simulink model "DTMF_DSK6713"  (Simulink 6.5)
settings: Solver=FixedStepDiscrete  StartTime=0  StopTime=20  RelTol=1e-3
PreLoadFcn:
  | Framesize=256,Fs=8192
values from neighbouring files (symbols this model uses):
  x = single(get(hObject,'Value'))    [AM.m]
undefined symbols (not defined in the file or in its folder): bit, dfilt, Fs
libraries: dspddes3 x14, dspobslib x3, commutil2 x2, c6713dsklib x1, c6000tgtpreflib x1, dsparch3 x1, dspswit3 x1, dspbuff3 x1, dsparch4 x1, rtdxBlocks x1
settings Model: Creator=stuartm  LastModifiedBy=dsp  ExtModeTrigMode=oneshot  ExtModeArmWhenConnect=off  BufferReuse=off  ProdHWDeviceType=TI C6000
settings SolverCC: PositivePriorityOrder=on
settings DataIOCC: LimitDataPoints=off  SaveOutput=off  SaveTime=off  SignalLoggingName=sigsOut
settings OptimizationCC: BlockReduction=off  BooleanDataType=off  OptimizeBlockIOStorage=off  BufferReuse=off  EnforceIntegerDowncast=off  ExpressionFolding=off  FoldNonRolledExpr=off  LocalBlockOutputs=off  OptimizeModelRefInitCode=on
settings DebuggingCC: SolverPrmCheckMsg=none  MultiTaskDSMMsg=warning  MultiTaskCondExecSysMsg=none  StrictBusMsg=None
settings HardwareCC: ProdBitPerLong=40  ProdIntDivRoundTo=Zero  ProdEndianess=LittleEndian  ProdHWDeviceType=TI C6000
settings RTWCC: SystemTargetFile=ti_c6000_ert.tlc  GenCodeOnly=on  TemplateMakefile=ti_c6000_ert.tmf  Description=Embedded Target for TI C6000 DSP (ERT)  ProcessScript=ti_c6000_ert_make_rtw_hook  IncludeERTFirstTime=on
settings CodeAppCC: IgnoreCustomStorageClasses=off
settings C6000ERTTargetCC: TargetFcnLib=ansi_tfl_tmw.mat  GenFloatMathFcnCalls=ANSI_C  UtilityFuncGeneration=Auto  GenerateFullHeader=on  GenerateSampleERTMain=off  GenerateTestInterfaces=off  IsPILTarget=off  ModelReferenceCompliant=on  IncludeMdlTerminateFcn=on  CombineOutputUpdateFcns=on  SuppressErrorStatus=off  IncludeFileDelimiter=Auto  ERTCustomFileBanners=on  SupportAbsoluteTime=on  LogVarNameModifier=rt_  MatFileLogging=off  MultiInstanceERTCode=off  SupportNonFinite=on  SupportComplex=on  PurelyIntegerCode=off  SupportContinuousTime=off  SupportNonInlinedSFcns=off  EnableShiftOperators=on  ParenthesesLevel=Nominal  GenerateErtSFunction=off  GenerateASAP2=off  ExtMode=off  ExtModeTransport=0  ExtModeStaticAlloc=off  ExtModeStaticAllocSize=1000000  ExtModeTesting=off  ExtModeMexFile=ext_comm  InlinedParameterPlacement=NonHierarchical  TargetOS=BareBoardExample  MultiInstanceErrorCode=Error  RateGroupingCode=on  RootIOFormat=Individual arguments  RTWCAPISignals=off  RTWCAPIParams=off  RTWCAPIStates=off  ERTSrcFileBannerTemplate=ert_code_template.cgt  ERTHdrFileBannerTemplate=ert_code_template.cgt  ERTDataSrcFileTemplate=ert_code_template.cgt  ERTDataHdrFileTemplate=ert_code_template.cgt  ERTCustomFileTemplate=example_file_process.tlc  ModuleNamingRule=Unspecified  SignalDisplayLevel=10  ParamTuneLevel=10  GlobalDataDefinition=Auto  DataDefinitionFile=global.c  GlobalDataReference=Auto  DataReferenceFile=global.h  GRTInterface=off  EnableUserReplacementTypes=off  MemSecPackage=--- None ---  MemSecDataConstants=Default  MemSecDataIO=Default  MemSecDataInternal=Default  MemSecDataParameters=Default  MemSecFuncInitTerm=Default  MemSecFuncExecute=Default  exportCCSObj=on  ccsObjName=CCS_Obj  useDSPBIOS=on  ProfileGenCode=on  InlineDSPBlks=on  FPopt=off  memModel=Far_Aggregate  optLevel=Function(-o2)  CompilerVerbosity=Quiet  InterruptThreshOnC6x=off  SymbolicDebugOnC6x=off  RetainAsmFiles=off  RetainObjFiles=on  CreateMapFile=on  UserStackSize=8192  c6000BuildAction=Build  OverrunAction=Notify_and_continue  OverrunNotificationMethod=Turn_on_LEDs

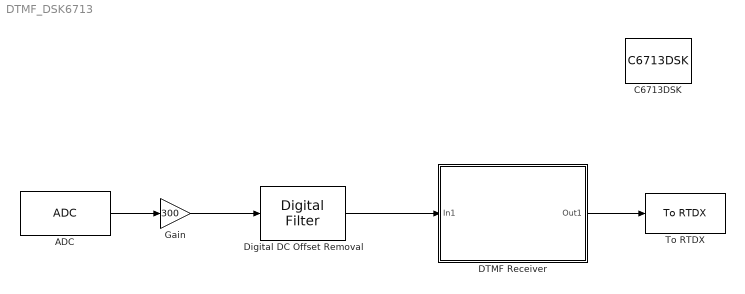
== system DTMF_DSK6713 ==
  ADC : c6713dsklib/ADC  ADCsource=Line In  MicGain=off  Stereo=off  SampleRate=8 kHz  CodecDataFormat=16-bit  OutputDataType=Double  Scaling=Normalize  SourceGain=0.0  FrameSize=256  inheritSampleTime=off
  C6713DSK : c6000tgtpreflib/C6713DSK  Tag=C6000 TARGET PREFERENCES BLOCK  SystemSampleTime=-1
  DTMF Receiver : Subsystem
  Digital DC Offset Removal : dsparch4/Digital Filter  DialogController=dspdialog.DigitalFilter  DialogControllerArgs=DataTag1  TypePopup=FIR (all zeros)  IIRFiltStruct=Direct form II transposed  AllPoleFiltStruct=Direct form  FIRFiltStruct=Direct form  CoeffSource=Specify via dialog  NumCoeffs=[0.5 -0.5]  DenCoeffs=[1 0.1]  BiQuadCoeffs=[1 0.3 0.4 1 0.1 0.2]  LatticeCoeffs=[0.2 0.4]  denIgnore=on  FiltPerSampPopup=One filter per frame  IC=0  ICnum=0  ICden=0  roundingMode=Floor  overflowMode=off  ScaleValues=1  scaleValueFracLength=14  stageInFracLength=15  stageOutFracLength=15  FilterSource=Specify via dialog  dfiltObjectName=dfilt.dffir([1 2 1])
  Gain : Gain  Gain=300
  To RTDX : rtdxBlocks/To RTDX  channelNameStr=OutputDigit  isBlocking=on  isChannelEnabled=on
  wires:
  Digital DC Offset Removal/1 -> DTMF Receiver/1(In1)
  DTMF Receiver/1(Out1) -> To RTDX/1
  Gain/1 -> Digital DC Offset Removal/1
  ADC/1 -> Gain/1

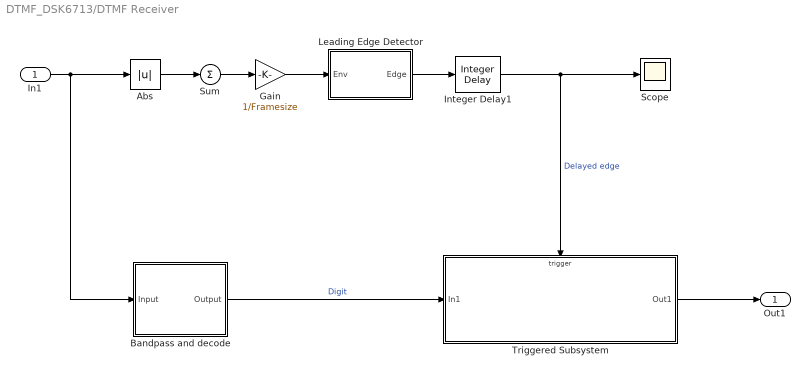
== system DTMF_DSK6713/DTMF Receiver ==
  In1 : Inport
  Abs : Abs  SaturateOnIntegerOverflow=on  SampleTime=-1
  Bandpass and decode : Subsystem
  Gain : Gain  Gain=1/Framesize  SaturateOnIntegerOverflow=on
  Integer Delay1 : dspobslib/Integer Delay  delay=1  ic=0  reset_popup=None
  Leading Edge Detector : Subsystem
  Scope : Scope
  Sum : Sum  Inputs=1  SaturateOnIntegerOverflow=on  InputSameDT=on
  Triggered Subsystem : Subsystem  TreatAsAtomicUnit=on
  Out1 : Outport
  wires:
  In1/1 -> Abs/1, Bandpass and decode/1(Input)
  Abs/1 -> Sum/1
  Sum/1 -> Gain/1
  Gain/1 -> Leading Edge Detector/1(Env)
  Triggered Subsystem/1(Out1) -> Out1/1
  Integer Delay1/1 -> Scope/1, Triggered Subsystem/Trigger  "Delayed edge"
  Bandpass and decode/1(Output) -> Triggered Subsystem/1(In1)  "Digit"
  Leading Edge Detector/1(Edge) -> Integer Delay1/1

== system DTMF_DSK6713/DTMF Receiver/Bandpass and decode ==
  Input : Inport
  Calculate Digit : Lookup2D  RowIndex=[1:4]  ColumnIndex=[1:3]  OutputValues=[1 2 3;4 5 6;7 8 9;10 0 11]  LookUpMeth=Use Input Nearest  OutDataTypeMode=double  SaturateOnIntegerOverflow=on  InputSameDT=on
  Calculate Column : Subsystem
  Calculate Row : Subsystem
  Output : Outport
  wires:
  Input/1 -> Calculate Column/1(In1), Calculate Row/1(In1)  "Input Tones"
  Calculate Digit/1 -> Output/1
  Calculate Row/1(Out1) -> Calculate Digit/1
  Calculate Column/1(Out1) -> Calculate Digit/2

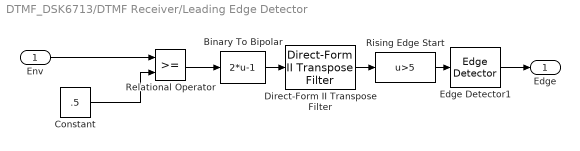
== system DTMF_DSK6713/DTMF Receiver/Leading Edge Detector ==
  Env : Inport
  Binary To Bipolar : Fcn  Expr=2*u-1
  Constant : Constant  Value=.5  OutDataType=sfix(16)  ConRadixGroup=Use specified scaling  OutScaling=2^0  SampleTime=inf  FramePeriod=inf
  Direct-Form II Transpose Filter : dsparch3/Direct-Form II Transpose Filter  num=[ones(1,4) -ones(1,4)]  den=1  ic=0
  Edge Detector1 : dspswit3/Edge Detector  SystemSampleTime=-1
  Relational Operator : RelationalOperator  InputSameDT=on
  Rising Edge Start : Fcn  Expr=u>5
  Edge : Outport  InitialOutput=0
  wires:
  Edge Detector1/1 -> Edge/1
  Direct-Form II Transpose Filter/1 -> Rising Edge Start/1
  Binary To Bipolar/1 -> Direct-Form II Transpose Filter/1
  Rising Edge Start/1 -> Edge Detector1/1
  Env/1 -> Relational Operator/1
  Constant/1 -> Relational Operator/2
  Relational Operator/1 -> Binary To Bipolar/1

== system DTMF_DSK6713/DTMF Receiver/Triggered Subsystem ==
  In1 : Inport
  Trigger : TriggerPort
  Buffer : dspbuff3/Buffer  N=11  V=10  ic=0
  Out1 : Outport
  wires:
  In1/1 -> Buffer/1
  Buffer/1 -> Out1/1

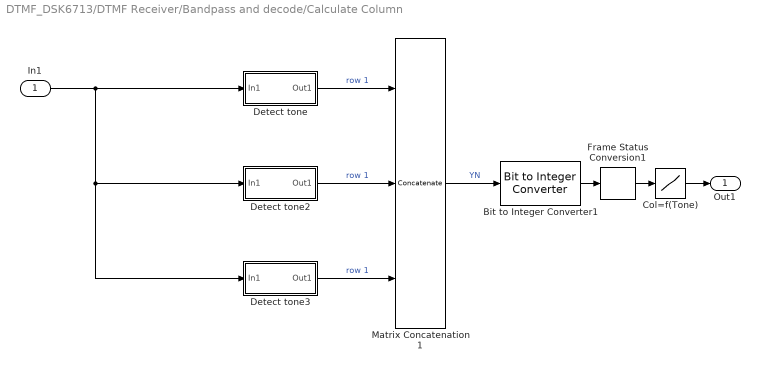
== system DTMF_DSK6713/DTMF Receiver/Bandpass and decode/Calculate Column ==
  In1 : Inport
  Bit to Integer Converter1 : commutil2/Bit to Integer Converter  nbits=3  outDtype=Same as input
  Col=f(Tone) : Lookup  InputValues=[0:7]  OutputValues=[0 1 2 0 3 0 0 0]  LookUpMeth=Use Input Nearest  OutDataType=sfix(16)  OutScaling=2^0  SaturateOnIntegerOverflow=on  SampleTime=-1  LUTDesignTableMode=Redesign Table  LUTDesignDataSource=Block Dialog  LUTDesignFunctionName=sqrt(x)  LUTDesignUseExistingBP=on  LUTDesignRelError=0.01  LUTDesignAbsError=1e-6  RndMeth=Floor
      settings: LockScale=off
  Detect tone : Subsystem  mask{Fs=Fs, F=1477}
      mask prompts: Fs "Sample Rate (Hz)"; F "Frequency"
      settings: AttributesFormatString=%<F> Hz
  Detect tone2 : Subsystem  mask{Fs=Fs, F=1336}
      mask prompts: Fs "Sample Rate (Hz)"; F "Frequency"
      settings: AttributesFormatString=%<F> Hz
  Detect tone3 : Subsystem  mask{Fs=Fs, F=1209}
      mask prompts: Fs "Sample Rate (Hz)"; F "Frequency"
      settings: AttributesFormatString=%<F> Hz
  Frame Status Conversion1 : dspobslib/Frame Status Conversion  SystemSampleTime=-1  growRefPort=off  outframe=Sample-based
  Matrix Concatenation1 : Concatenate  NumInputs=3  Mode=Vertical matrix concatenation
  Out1 : Outport
  wires:
  Matrix Concatenation1/1 -> Bit to Integer Converter1/1  "YN"
  Bit to Integer Converter1/1 -> Frame Status Conversion1/1
  Frame Status Conversion1/1 -> Col=f(Tone)/1
  Detect tone/1(Out1) -> Matrix Concatenation1/1  "row 1"
  Detect tone2/1(Out1) -> Matrix Concatenation1/2  "row 1"
  Detect tone3/1(Out1) -> Matrix Concatenation1/3  "row 1"
  In1/1 -> Detect tone2/1(In1), Detect tone3/1(In1), Detect tone/1(In1)
  Col=f(Tone)/1 -> Out1/1

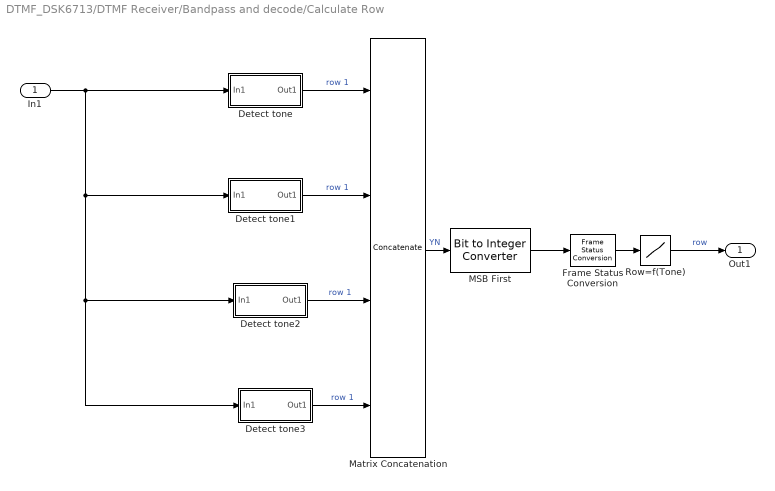
== system DTMF_DSK6713/DTMF Receiver/Bandpass and decode/Calculate Row ==
  In1 : Inport
  Detect tone : Subsystem  mask{Fs=Fs, F=941}
      mask prompts: Fs "Sample Rate (Hz)"; F "Frequency"
      settings: AttributesFormatString=%<F> Hz
  Detect tone1 : Subsystem  mask{Fs=Fs, F=852}
      mask prompts: Fs "Sample Rate (Hz)"; F "Frequency"
      settings: AttributesFormatString=%<F> Hz
  Detect tone2 : Subsystem  mask{Fs=Fs, F=770}
      mask prompts: Fs "Sample Rate (Hz)"; F "Frequency"
      settings: AttributesFormatString=%<F> Hz
  Detect tone3 : Subsystem  mask{Fs=Fs, F=697}
      mask prompts: Fs "Sample Rate (Hz)"; F "Frequency"
      settings: AttributesFormatString=%<F> Hz
  Frame Status Conversion : dspobslib/Frame Status Conversion  SystemSampleTime=-1  growRefPort=off  outframe=Sample-based
  MSB First : commutil2/Bit to Integer Converter  nbits=4  outDtype=Same as input
  Matrix Concatenation : Concatenate  NumInputs=4  Mode=Vertical matrix concatenation
  Row=f(Tone) : Lookup  InputValues=[0:15]  OutputValues=[0 1 2 0 3 0 0 0 4 0 0 0 0 0 0 0]  LookUpMeth=Use Input Nearest  OutDataType=sfix(16)  OutScaling=2^0  SaturateOnIntegerOverflow=on  SampleTime=-1  LUTDesignTableMode=Redesign Table  LUTDesignDataSource=Block Dialog  LUTDesignFunctionName=sqrt(x)  LUTDesignUseExistingBP=on  LUTDesignRelError=0.01  LUTDesignAbsError=1e-6  RndMeth=Floor
      settings: LockScale=off
  Out1 : Outport
  wires:
  Detect tone/1(Out1) -> Matrix Concatenation/1  "row 1"
  Matrix Concatenation/1 -> MSB First/1  "YN"
  MSB First/1 -> Frame Status Conversion/1
  Frame Status Conversion/1 -> Row=f(Tone)/1
  Detect tone1/1(Out1) -> Matrix Concatenation/2  "row 1"
  Detect tone2/1(Out1) -> Matrix Concatenation/3  "row 1"
  Detect tone3/1(Out1) -> Matrix Concatenation/4  "row 1"
  In1/1 -> Detect tone/1(In1), Detect tone1/1(In1), Detect tone2/1(In1), Detect tone3/1(In1)
  Row=f(Tone)/1 -> Out1/1  "row"

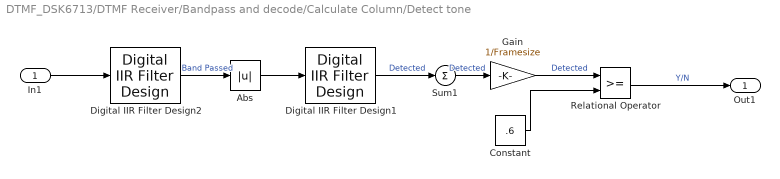
== system DTMF_DSK6713/DTMF Receiver/Bandpass and decode/Calculate Column/Detect tone ==
  In1 : Inport
  Abs : Abs  SaturateOnIntegerOverflow=on  SampleTime=-1
  Constant : Constant  Value=.6  OutDataType=sfix(16)  ConRadixGroup=Use specified scaling  OutScaling=2^0  SampleTime=inf  FramePeriod=inf
  Digital IIR Filter Design1 : dspddes3/Digital IIR Filter Design  SystemSampleTime=-1  method=Butterworth  filttype=Lowpass  N=4  Wlo=100/(Fs/2)  Whi=(F+10)/(Fs/2)  Rp=1  Rs=20
  Digital IIR Filter Design2 : dspddes3/Digital IIR Filter Design  SystemSampleTime=-1  method=Chebyshev I  filttype=Bandpass  N=4  Wlo=(F-10)/(Fs/2)  Whi=(F+10)/(Fs/2)  Rp=1  Rs=20
  Gain : Gain  Gain=1/Framesize  SaturateOnIntegerOverflow=on
  Relational Operator : RelationalOperator  InputSameDT=on
  Sum1 : Sum  Inputs=1  SaturateOnIntegerOverflow=on  InputSameDT=on
  Out1 : Outport
  wires:
  Digital IIR Filter Design1/1 -> Sum1/1  "Detected"
  Relational Operator/1 -> Out1/1  "Y/N"
  Constant/1 -> Relational Operator/2
  Abs/1 -> Digital IIR Filter Design1/1
  Digital IIR Filter Design2/1 -> Abs/1  "Band Passed"
  In1/1 -> Digital IIR Filter Design2/1
  Sum1/1 -> Gain/1  "Detected"
  Gain/1 -> Relational Operator/1  "Detected"

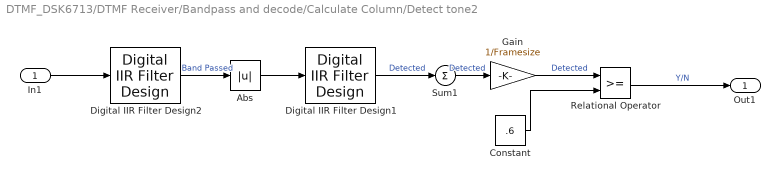
== system DTMF_DSK6713/DTMF Receiver/Bandpass and decode/Calculate Column/Detect tone2 ==
  In1 : Inport
  Abs : Abs  SaturateOnIntegerOverflow=on  SampleTime=-1
  Constant : Constant  Value=.6  OutDataType=sfix(16)  ConRadixGroup=Use specified scaling  OutScaling=2^0  SampleTime=inf  FramePeriod=inf
  Digital IIR Filter Design1 : dspddes3/Digital IIR Filter Design  SystemSampleTime=-1  method=Butterworth  filttype=Lowpass  N=4  Wlo=100/(Fs/2)  Whi=(F+10)/(Fs/2)  Rp=1  Rs=20
  Digital IIR Filter Design2 : dspddes3/Digital IIR Filter Design  SystemSampleTime=-1  method=Chebyshev I  filttype=Bandpass  N=4  Wlo=(F-10)/(Fs/2)  Whi=(F+10)/(Fs/2)  Rp=1  Rs=20
  Gain : Gain  Gain=1/Framesize  SaturateOnIntegerOverflow=on
  Relational Operator : RelationalOperator  InputSameDT=on
  Sum1 : Sum  Inputs=1  SaturateOnIntegerOverflow=on  InputSameDT=on
  Out1 : Outport
  wires:
  Gain/1 -> Relational Operator/1  "Detected"
  Sum1/1 -> Gain/1  "Detected"
  In1/1 -> Digital IIR Filter Design2/1
  Digital IIR Filter Design2/1 -> Abs/1  "Band Passed"
  Abs/1 -> Digital IIR Filter Design1/1
  Constant/1 -> Relational Operator/2
  Relational Operator/1 -> Out1/1  "Y/N"
  Digital IIR Filter Design1/1 -> Sum1/1  "Detected"

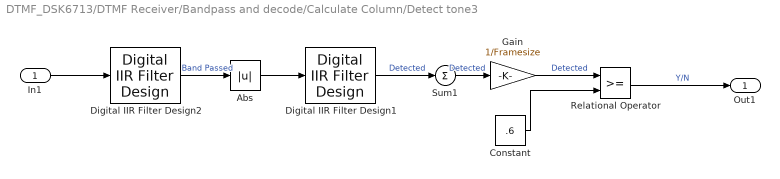
== system DTMF_DSK6713/DTMF Receiver/Bandpass and decode/Calculate Column/Detect tone3 ==
  In1 : Inport
  Abs : Abs  SaturateOnIntegerOverflow=on  SampleTime=-1
  Constant : Constant  Value=.6  OutDataType=sfix(16)  ConRadixGroup=Use specified scaling  OutScaling=2^0  SampleTime=inf  FramePeriod=inf
  Digital IIR Filter Design1 : dspddes3/Digital IIR Filter Design  SystemSampleTime=-1  method=Butterworth  filttype=Lowpass  N=4  Wlo=100/(Fs/2)  Whi=(F+10)/(Fs/2)  Rp=1  Rs=20
  Digital IIR Filter Design2 : dspddes3/Digital IIR Filter Design  SystemSampleTime=-1  method=Chebyshev I  filttype=Bandpass  N=4  Wlo=(F-10)/(Fs/2)  Whi=(F+10)/(Fs/2)  Rp=1  Rs=20
  Gain : Gain  Gain=1/Framesize  SaturateOnIntegerOverflow=on
  Relational Operator : RelationalOperator  InputSameDT=on
  Sum1 : Sum  Inputs=1  SaturateOnIntegerOverflow=on  InputSameDT=on
  Out1 : Outport
  wires:
  Digital IIR Filter Design1/1 -> Sum1/1  "Detected"
  Relational Operator/1 -> Out1/1  "Y/N"
  Constant/1 -> Relational Operator/2
  Abs/1 -> Digital IIR Filter Design1/1
  Digital IIR Filter Design2/1 -> Abs/1  "Band Passed"
  In1/1 -> Digital IIR Filter Design2/1
  Sum1/1 -> Gain/1  "Detected"
  Gain/1 -> Relational Operator/1  "Detected"

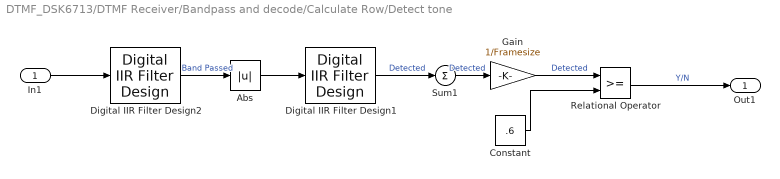
== system DTMF_DSK6713/DTMF Receiver/Bandpass and decode/Calculate Row/Detect tone ==
  In1 : Inport
  Abs : Abs  SaturateOnIntegerOverflow=on  SampleTime=-1
  Constant : Constant  Value=.6  OutDataType=sfix(16)  ConRadixGroup=Use specified scaling  OutScaling=2^0  SampleTime=inf  FramePeriod=inf
  Digital IIR Filter Design1 : dspddes3/Digital IIR Filter Design  SystemSampleTime=-1  method=Butterworth  filttype=Lowpass  N=4  Wlo=100/(Fs/2)  Whi=(F+10)/(Fs/2)  Rp=1  Rs=20
  Digital IIR Filter Design2 : dspddes3/Digital IIR Filter Design  SystemSampleTime=-1  method=Chebyshev I  filttype=Bandpass  N=4  Wlo=(F-10)/(Fs/2)  Whi=(F+10)/(Fs/2)  Rp=1  Rs=20
  Gain : Gain  Gain=1/Framesize  SaturateOnIntegerOverflow=on
  Relational Operator : RelationalOperator  InputSameDT=on
  Sum1 : Sum  Inputs=1  SaturateOnIntegerOverflow=on  InputSameDT=on
  Out1 : Outport
  wires:
  Gain/1 -> Relational Operator/1  "Detected"
  Sum1/1 -> Gain/1  "Detected"
  In1/1 -> Digital IIR Filter Design2/1
  Digital IIR Filter Design2/1 -> Abs/1  "Band Passed"
  Abs/1 -> Digital IIR Filter Design1/1
  Constant/1 -> Relational Operator/2
  Relational Operator/1 -> Out1/1  "Y/N"
  Digital IIR Filter Design1/1 -> Sum1/1  "Detected"

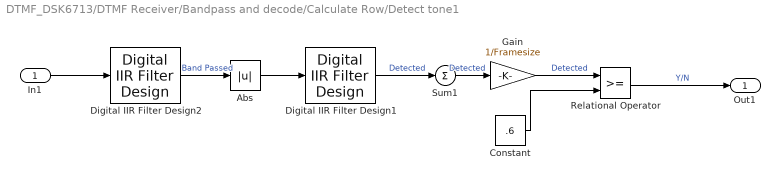
== system DTMF_DSK6713/DTMF Receiver/Bandpass and decode/Calculate Row/Detect tone1 ==
  In1 : Inport
  Abs : Abs  SaturateOnIntegerOverflow=on  SampleTime=-1
  Constant : Constant  Value=.6  OutDataType=sfix(16)  ConRadixGroup=Use specified scaling  OutScaling=2^0  SampleTime=inf  FramePeriod=inf
  Digital IIR Filter Design1 : dspddes3/Digital IIR Filter Design  SystemSampleTime=-1  method=Butterworth  filttype=Lowpass  N=4  Wlo=100/(Fs/2)  Whi=(F+10)/(Fs/2)  Rp=1  Rs=20
  Digital IIR Filter Design2 : dspddes3/Digital IIR Filter Design  SystemSampleTime=-1  method=Chebyshev I  filttype=Bandpass  N=4  Wlo=(F-10)/(Fs/2)  Whi=(F+10)/(Fs/2)  Rp=1  Rs=20
  Gain : Gain  Gain=1/Framesize  SaturateOnIntegerOverflow=on
  Relational Operator : RelationalOperator  InputSameDT=on
  Sum1 : Sum  Inputs=1  SaturateOnIntegerOverflow=on  InputSameDT=on
  Out1 : Outport
  wires:
  Digital IIR Filter Design1/1 -> Sum1/1  "Detected"
  Relational Operator/1 -> Out1/1  "Y/N"
  Constant/1 -> Relational Operator/2
  Abs/1 -> Digital IIR Filter Design1/1
  Digital IIR Filter Design2/1 -> Abs/1  "Band Passed"
  In1/1 -> Digital IIR Filter Design2/1
  Sum1/1 -> Gain/1  "Detected"
  Gain/1 -> Relational Operator/1  "Detected"

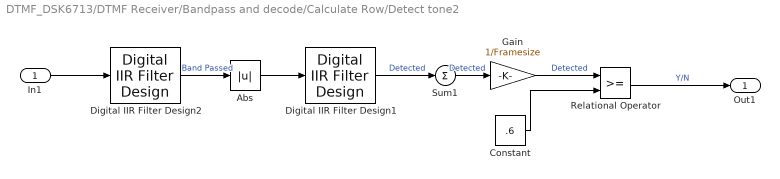
== system DTMF_DSK6713/DTMF Receiver/Bandpass and decode/Calculate Row/Detect tone2 ==
  In1 : Inport
  Abs : Abs  SaturateOnIntegerOverflow=on  SampleTime=-1
  Constant : Constant  Value=.6  OutDataType=sfix(16)  ConRadixGroup=Use specified scaling  OutScaling=2^0  SampleTime=inf  FramePeriod=inf
  Digital IIR Filter Design1 : dspddes3/Digital IIR Filter Design  SystemSampleTime=-1  method=Butterworth  filttype=Lowpass  N=4  Wlo=100/(Fs/2)  Whi=(F+10)/(Fs/2)  Rp=1  Rs=20
  Digital IIR Filter Design2 : dspddes3/Digital IIR Filter Design  SystemSampleTime=-1  method=Chebyshev I  filttype=Bandpass  N=4  Wlo=(F-10)/(Fs/2)  Whi=(F+10)/(Fs/2)  Rp=1  Rs=20
  Gain : Gain  Gain=1/Framesize  SaturateOnIntegerOverflow=on
  Relational Operator : RelationalOperator  InputSameDT=on
  Sum1 : Sum  Inputs=1  SaturateOnIntegerOverflow=on  InputSameDT=on
  Out1 : Outport
  wires:
  Gain/1 -> Relational Operator/1  "Detected"
  Sum1/1 -> Gain/1  "Detected"
  In1/1 -> Digital IIR Filter Design2/1
  Digital IIR Filter Design2/1 -> Abs/1  "Band Passed"
  Abs/1 -> Digital IIR Filter Design1/1
  Constant/1 -> Relational Operator/2
  Relational Operator/1 -> Out1/1  "Y/N"
  Digital IIR Filter Design1/1 -> Sum1/1  "Detected"

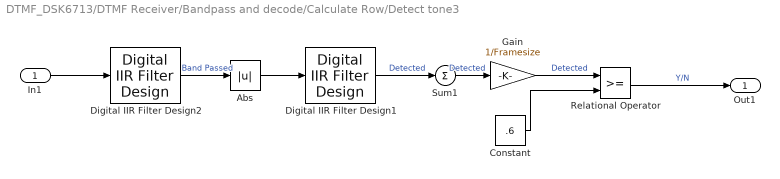
== system DTMF_DSK6713/DTMF Receiver/Bandpass and decode/Calculate Row/Detect tone3 ==
  In1 : Inport
  Abs : Abs  SaturateOnIntegerOverflow=on  SampleTime=-1
  Constant : Constant  Value=.6  OutDataType=sfix(16)  ConRadixGroup=Use specified scaling  OutScaling=2^0  SampleTime=inf  FramePeriod=inf
  Digital IIR Filter Design1 : dspddes3/Digital IIR Filter Design  SystemSampleTime=-1  method=Butterworth  filttype=Lowpass  N=4  Wlo=100/(Fs/2)  Whi=(F+10)/(Fs/2)  Rp=1  Rs=20
  Digital IIR Filter Design2 : dspddes3/Digital IIR Filter Design  SystemSampleTime=-1  method=Chebyshev I  filttype=Bandpass  N=4  Wlo=(F-10)/(Fs/2)  Whi=(F+10)/(Fs/2)  Rp=1  Rs=20
  Gain : Gain  Gain=1/Framesize  SaturateOnIntegerOverflow=on
  Relational Operator : RelationalOperator  InputSameDT=on
  Sum1 : Sum  Inputs=1  SaturateOnIntegerOverflow=on  InputSameDT=on
  Out1 : Outport
  wires:
  Digital IIR Filter Design1/1 -> Sum1/1  "Detected"
  Relational Operator/1 -> Out1/1  "Y/N"
  Constant/1 -> Relational Operator/2
  Abs/1 -> Digital IIR Filter Design1/1
  Digital IIR Filter Design2/1 -> Abs/1  "Band Passed"
  In1/1 -> Digital IIR Filter Design2/1
  Sum1/1 -> Gain/1  "Detected"
  Gain/1 -> Relational Operator/1  "Detected"
